simulink model "wastegateflow"  (R2013a)
settings: Solver=ode45  StartTime=0.0  StopTime=10.0  RelTol=1e-3
values from neighbouring files (symbols this model uses):
  R_exh = 280    [Init_Project1.m]
  T_em = mean(T_em)    [Init_Project1.m]    (also in Init_Project2.m = mean(T_t*(1-eta_T.*(1-Pi_T.^((gamma_exh-1)/gamma_exh)))))
settings Model: Creator=rasme879  LastModifiedBy=rasme879

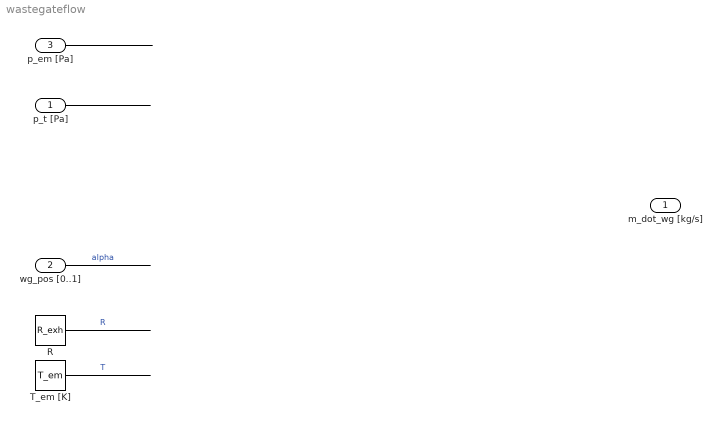
== system wastegateflow ==
  p_t [Pa] : Inport
  wg_pos [0..1] : Inport  Port=2
  p_em [Pa] : Inport  Port=3
  R : Constant  Value=R_exh
  T_em [K] : Constant  Value=T_em
  m_dot_wg [kg/s] : Outport
  wires:
  p_em [Pa]/1 -> ?
  p_t [Pa]/1 -> ?
  wg_pos [0..1]/1 -> ?  "alpha"
  R/1 -> ?  "R"
  T_em [K]/1 -> ?  "T"
  ? -> m_dot_wg [kg/s]/1
